simulink model "untitled"  (R2020a)
settings: Solver=VariableStepAuto  StartTime=2.353  StopTime=3.9  FixedStep=1e-2  MaxStep=1e-2  RelTol=1e-3
values from neighbouring files (symbols this model uses):
  denom_cheby = [1 -0.613126393211 0.273045514473]    [MOTORKENNLINIE.mat]    (also in kennlinie_und_modell.mat; matlab.mat; neuedaten.mat; neuedaten2.mat)
  denum = [1 -1.14298050254 0.412801598096]    [MOTORKENNLINIE.mat]    (also in kennlinie_und_modell.mat; matlab.mat; neuedaten.mat; neuedaten2.mat)
  num = [0.0674552738891 0.134910547778 0.0674552738891]    [MOTORKENNLINIE.mat]    (also in kennlinie_und_modell.mat; matlab.mat; neuedaten.mat; neuedaten2.mat)
  num_cheby = [0.163091272387 0.326182544774 0.163091272387]    [MOTORKENNLINIE.mat]    (also in kennlinie_und_modell.mat; matlab.mat; neuedaten.mat; neuedaten2.mat)
undefined symbols (not defined in the file or in its folder): Discrete, Time
libraries: ctrlSharedLib x1

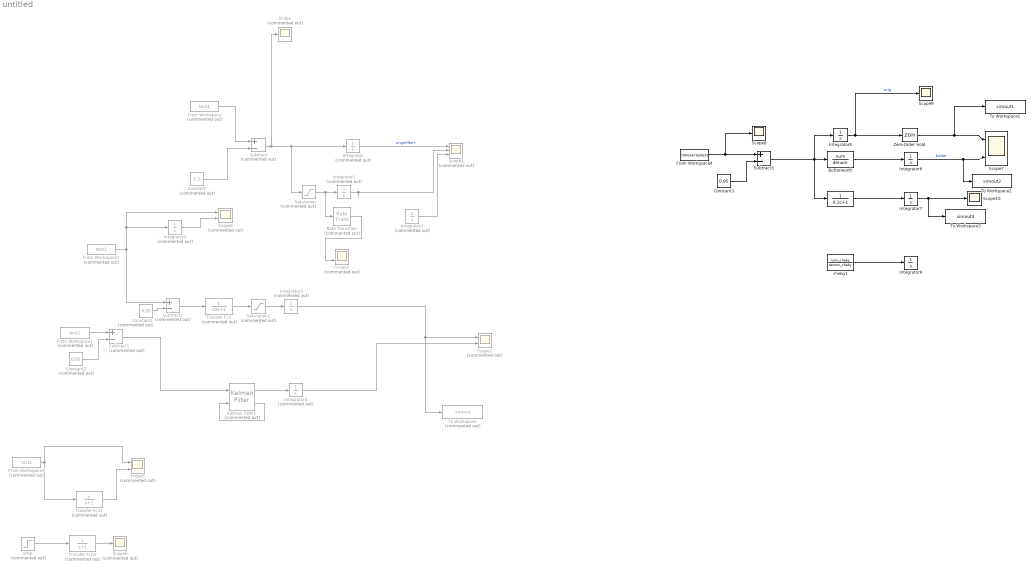
== system untitled ==
  " " : TransferFcn  Numerator=1  Denominator=[0.1 1]
  "Butterworth " : DiscreteTransferFcn  Numerator=num  Denominator=denum
  Constant : Constant  Commented=on  Value=1.2
  Constant1 : Constant  Commented=on  Value=0.95
  Constant2 : Constant  Commented=on  Value=0.95
  Constant3 : Constant  Value=0.95
  From Workspace{,1..3} (4 alike) : FromWorkspace  Commented=on  VariableName=test1  SampleTime=-1  Interpolate=off  OutputAfterFinalValue=Holding final value
  From Workspace4 : FromWorkspace  VariableName=timeseriestest  SampleTime=-1  Interpolate=off  OutputAfterFinalValue=Holding final value
  Integrator{,1..5} (6 alike) : Integrator  Commented=on
  Integrator{6..9} (4 alike) : Integrator
  Kalman Filter1 : ctrlSharedLib/Kalman Filter  Commented=on  TimeDomain=Discrete-Time  UseCurrentEstimator=on  ModelSource=LTI State-Space Variable  ModelSourceVariable=ss(0.95,1,1,0,1)  A=0.95  B=1  C=1  D=0  NumberOfStates=1  NumberOfInputs=1  NumberOfOutputs=1  InitialEstimateSource=Dialog  X0=0  P0=10  UseK=off  UseGH=off  NumberOfProcessNoiseInputs=1  G=1  TimeInvariantG=on  H=0  TimeInvariantH=on  Q=0.05  TimeInvariantQ=on  R=1  TimeInvariantR=on  N=0  TimeInvariantN=on  AddInputPort=on  AddEnablePort=off  OutputEstimatedY=on  OutputP=off  Ts=-1
  Rate Transition : RateTransition  Commented=on  OutPortSampleTime=0.001
  Saturation : Saturate  Commented=on  UpperLimit=inf  LowerLimit=0
  Saturation2 : Saturate  Commented=on  UpperLimit=inf  LowerLimit=-inf
  Scope : Scope  Commented=on
  Scope1 : Scope  Commented=on  NumInputPorts=3
  Scope10 : Scope
  Scope{2..5} (4 alike) : Scope  Commented=on  NumInputPorts=2
  Scope6 : Scope  Commented=on
  Scope7 : Scope  NumInputPorts=2
  Scope8 : Scope
  Scope9 : Scope
  Step : Step  Commented=on  SampleTime=0
  Subtract : Sum  Commented=on  Inputs=+-
  Subtract1 : Sum  Commented=on  Inputs=+-
  Subtract2 : Sum  Commented=on  Inputs=+-
  Subtract3 : Sum  Inputs=+-
  To Workspace : ToWorkspace  Commented=on  VariableName=simout  SaveFormat=Timeseries  SampleTime=-1
  To Workspace1 : ToWorkspace  VariableName=simout1  SampleTime=-1
  To Workspace2 : ToWorkspace  VariableName=simout2  SampleTime=-1
  To Workspace3 : ToWorkspace  VariableName=simout3  SaveFormat=Timeseries  SampleTime=-1
  Transfer Fcn : TransferFcn  Commented=on  Denominator=[10 1]
  Transfer Fcn1 : TransferFcn  Commented=on  Numerator=[1 0]  Denominator=[1 1]
  Transfer Fcn2 : TransferFcn  Commented=on  Numerator=[1 0]  Denominator=[1 1]
  Zero-Order Hold : ZeroOrderHold  SampleTime=-1
  cheby1 : DiscreteTransferFcn  Numerator=num_cheby  Denominator=denom_cheby
  wires:
  Constant/1 -> Subtract/2
  From Workspace/1 -> Subtract/1
  Subtract/1 -> Saturation/1, Integrator/1, Scope/1
  Integrator/1 -> Scope1/1  "ungefiltert"
  Saturation/1 -> Rate Transition/1, Integrator1/1
  Integrator1/1 -> Scope1/2
  ? -> Integrator2/1
  Integrator2/1 -> Scope1/3
  Rate Transition/1 -> Scope2/2
  From Workspace1/1 -> Subtract1/1
  Integrator3/1 -> Scope3/1, To Workspace/1
  Kalman Filter1/2 -> Kalman Filter1/2
  Subtract1/1 -> Kalman Filter1/1
  Kalman Filter1/1 -> Integrator4/1
  Integrator4/1 -> Scope3/2
  Transfer Fcn/1 -> Saturation2/1
  Constant2/1 -> Subtract1/2
  From Workspace2/1 -> Integrator5/1, Scope4/1, Subtract2/1
  From Workspace3/1 -> Scope5/1, Transfer Fcn1/1
  Transfer Fcn1/1 -> Scope5/2
  Step/1 -> Transfer Fcn2/1
  Transfer Fcn2/1 -> Scope6/1
  Subtract2/1 -> Transfer Fcn/1
  Saturation2/1 -> Integrator3/1
  Integrator5/1 -> Scope4/2
  Constant1/1 -> Subtract2/2
  Constant3/1 -> Subtract3/2
  "Butterworth "/1 -> Integrator6/1
  Subtract3/1 -> " "/1, Integrator8/1, "Butterworth "/1
  Integrator6/1 -> To Workspace2/1, Scope7/2  "butter"
  " "/1 -> Integrator7/1
  Integrator8/1 -> Scope9/1, Zero-Order Hold/1  "orig"
  cheby1/1 -> Integrator9/1
  Zero-Order Hold/1 -> To Workspace1/1, Scope7/1
  From Workspace4/1 -> Scope8/1, Subtract3/1
  Integrator7/1 -> To Workspace3/1, Scope10/1
